simulink model "ptos_sim"  (Simulink 7.9)
settings: Solver=ode45  StartTime=0.0  StopTime=2.5*sqrt(r/N)  RelTol=1e-5
values from neighbouring files (symbols this model uses):
  k1 = signal1(2)    [f_ptos.m]    (also in fig10_05.m = [0, 0.4]; fig10_06.m = [0 .4]; fig10_15.m = [0:.001:1.4]; fig10_16.m = [0 .4])
  k2 = sqrt(2*k1/Na)    [f_ptos.m]    (also in fig10_15.m = [1.4:.00001:1.5])
  N = reshape(xx(n*nm+1:end),p,nm)    [Modelfollowingdesign.m]    (also in f_tos.m = 1; fig10_18.m = S\r; fig10_19.m = S\r; fig10_20.m = S\r)
  Na = signal1(1)    [f_ptos.m]
  r = rlocus(Aol,Bol,Col,Dol,k5)    [fig10_15.m]    (also in fig10_18.m = [0*B;1]; fig10_19.m = [0*B;1]; fig10_20.m = [0*B;1]; fig10_21.m = [0*B;1])
settings Model: Creator=abbas  LastModifiedBy=abbas
settings DataIOCC: SignalLoggingName=sigsOut
settings OptimizationCC: BooleanDataType=off  InlineParams=on  InlineInvariantSignals=on  InitFltsAndDblsToZero=on
settings DebuggingCC: SaveWithParameterizedLinksMsg=none  SignalResolutionControl=TryResolveAllWithWarning  SolverPrmCheckMsg=none  MultiTaskDSMMsg=warning  MultiTaskCondExecSysMsg=none  FcnCallInpInsideContextMsg=Use local settings  StrictBusMsg=None
settings HardwareCC: TargetUnknown=on
settings RTWCC: IncludeERTFirstTime=on
settings GRTTargetCC: TargetFcnLib=ansi_tfl_tmw.mat  CombineOutputUpdateFcns=off  GRTInterface=on

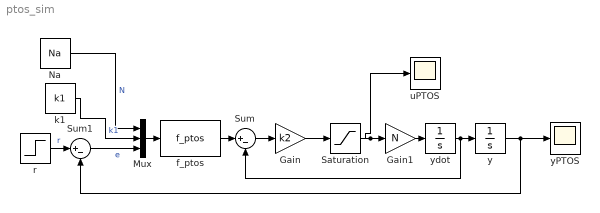
== system ptos_sim ==
  " f_ptos" : MATLABFcn  MATLABFcn=f_ptos  OutputDimensions=1
  " r" : Step  Time=0  After=r  SampleTime=0
  " ydot" : Integrator
  Gain : Gain  Gain=k2  SaturateOnIntegerOverflow=on  OutDataTypeStr=Inherit: Same as input  ParamDataTypeStr=Inherit: Same as input
  Gain1 : Gain  Gain=N  SaturateOnIntegerOverflow=on  OutDataTypeStr=Inherit: Same as input  ParamDataTypeStr=Inherit: Same as input
  Mux : Mux  Inputs=N,k1,e
  Na : Constant  Value=Na
  Saturation : Saturate  UpperLimit=1  LowerLimit=-1
  Sum : Sum  Inputs=|+-  SaturateOnIntegerOverflow=on  InputSameDT=on  OutDataTypeStr=Inherit: Same as first input
  Sum1 : Sum  Inputs=|+-  SaturateOnIntegerOverflow=on  InputSameDT=on  OutDataTypeStr=Inherit: Same as first input
  k1 : Constant  Value=k1
  uPTOS : Scope
      settings: YMin=-1.2  YMax=1.2  SaveName=uptos
  y : Integrator
  yPTOS : Scope
      settings: YMin=-0.1  YMax=1.1  SaveName=yptos
  wires:
  " ydot"/1 -> Sum/2, y/1
  Saturation/1 -> Gain1/1, uPTOS/1
  y/1 -> Sum1/2, yPTOS/1
  " r"/1 -> Sum1/1  "r"
  Gain/1 -> Saturation/1
  Sum/1 -> Gain/1
  Gain1/1 -> " ydot"/1
  " f_ptos"/1 -> Sum/1
  Mux/1 -> " f_ptos"/1
  Sum1/1 -> Mux/3  "e"
  Na/1 -> Mux/1  "N"
  k1/1 -> Mux/2  "k1"
